simulink model "Suspension_model_PID"  (R2023a)
settings: Solver=ode1  StartTime=0.0  StopTime=10  FixedStep=0.001  RelTol=1e-3
undefined symbols (not defined in the file or in its folder): A, B, C, D, k
libraries: slpidlib x1
settings Model: Creator=ku53058  LastModifiedBy=sevva
settings SolverCC: AlgebraicLoopSolver=TrustRegion
settings DataIOCC: ReturnWorkspaceOutputs=off
settings OptimizationCC: LifeSpan=inf
settings DebuggingCC: UnconnectedInputMsg=warning  UnconnectedOutputMsg=warning  UnconnectedLineMsg=warning  ArithmeticOperatorsInVariantConditions=warning
settings ModelReferenceCC: EnableRefExpFcnMdlSchedulingChecks=on
settings SFSimCC: SimUseLocalCustomCode=off  CustomCodeUndefinedFunction=UseInterfaceOnly
settings RTWCC: RTWUseLocalCustomCode=off
settings CodeAppCC: StateflowObjectComments=on

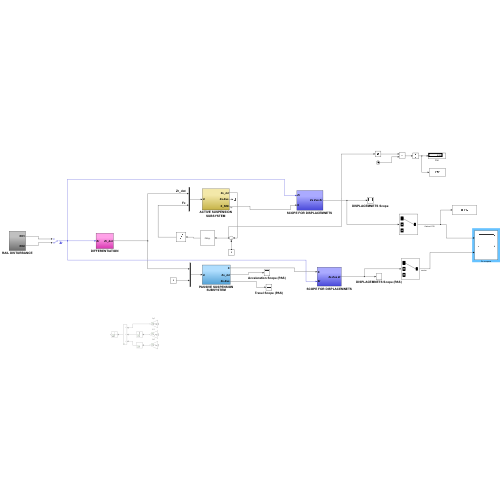
[thumbnail: Simulink's stored preview of the top-level diagram]
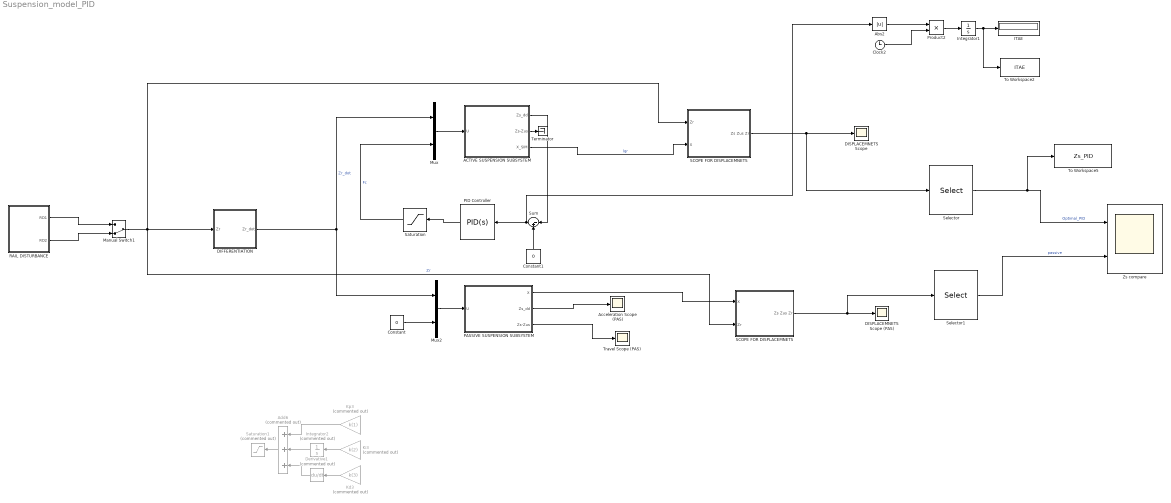
== system Suspension_model_PID ==
  ACTIVE SUSPENSION SUBSYSTEM : Subsystem
  Abs2 : Abs  SaturateOnIntegerOverflow=off
  Acceleration Scope (PAS) : Scope
  Add6 : Sum  Commented=on  Inputs=+++
  Clock2 : Clock
  Constant : Constant  Value=0
  Constant1 : Constant  Value=0
  DIFFERENTIATION : Subsystem
  DISPLACEMNETS Scope : Scope
  DISPLACEMNETS Scope (PAS) : Scope
  Derivative1 : Derivative  Commented=on
  ITAE : Display
  Integrator1 : Integrator
  Integrator2 : Integrator  Commented=on
  Kd3 : Gain  Commented=on  Gain=k(3)
  Ki3 : Gain  Commented=on  Gain=k(2)
  Kp3 : Gain  Commented=on  Gain=k(1)
  Manual Switch1 : ManualSwitch  CurrentSetting=0
  Mux : Mux  Inputs=2
  Mux2 : Mux  Inputs=2
  PASSIVE SUSPENSION SUBSYSTEM : Subsystem
  PID Controller : slpidlib/PID Controller  Controller=PID  Form=Parallel  TimeDomain=Continuous-time  UseExternalTs=off  SampleTime=-1  IntegratorMethod=Forward Euler  FilterMethod=Forward Euler  ControllerParametersSource=internal  P=150  I=3000  UseKiTs=off  D=45  N=100  UseFilter=on  TunerSelectOption=Transfer Function Based (PID Tuner App)  InitialConditionSource=internal  InitialConditionForIntegrator=0  InitialConditionForFilter=0  DifferentiatorICPrevScaledInput=0  ExternalReset=none  TrackingMode=off  Kt=1  LimitOutput=off  SatLimitsSource=internal  UpperSaturationLimit=inf  LowerSaturationLimit=-inf  LinearizeAsGain=on  AntiWindupMode=none  Kb=1  LimitIntegrator=off  UpperIntegratorSaturationLimit=inf  LowerIntegratorSaturationLimit=-inf  POutMin=[]  POutMax=[]  IOutMin=[]  IOutMax=[]  DOutMin=[]  DOutMax=[]  NOutMin=[]  NOutMax=[]  SumOutMin=[]  SumOutMax=[]  SaturationOutMin=[]  SaturationOutMax=[]  PParamMin=[]  PParamMax=[]  IParamMin=[]  IParamMax=[]  DParamMin=[]  DParamMax=[]  NParamMin=[]  NParamMax=[]  KbParamMin=[]  KbParamMax=[]  KtParamMin=[]  KtParamMax=[]  KbOutMin=[]  KbOutMax=[]  KtOutMin=[]  KtOutMax=[]  IntegratorOutMin=[]  IntegratorOutMax=[]  FilterOutMin=[]  FilterOutMax=[]  SumI1OutMin=[]  SumI1OutMax=[]  SumI2OutMin=[]  SumI2OutMax=[]  SumI3OutMin=[]  SumI3OutMax=[]  SumI4OutMin=[]  SumI4OutMax=[]  SumDOutMin=[]  SumDOutMax=[]  DifferentiatorOutMin=[]  DifferentiatorOutMax=[]  FilterDiffOutCoefMin=[]  FilterDiffOutCoefMax=[]  ReciprocalOutMin=[]  ReciprocalOutMax=[]  SumDenOutMin=[]  SumDenOutMax=[]  SumNumOutMin=[]  SumNumOutMax=[]  DivideOutMin=[]  DivideOutMax=[]  UdiffTsProdOutMin=[]  UdiffTsProdOutMax=[]  NTsProdOutMin=[]  NTsProdOutMax=[]  UintegralTsProdOutMin=[]  UintegralTsProdOutMax=[]  UngainTsProdOutMin=[]  UngainTsProdOutMax=[]  ClampingZeroOutDataTypeStr=Inherit: Inherit via back propagation  ClampingZeroOutMin=[]  ClampingZeroOutMax=[]  FilterDenConstantOutDataTypeStr=Inherit: Inherit via back propagation  FilterDenConstantOutMin=[]  FilterDenConstantOutMax=[]  PCopyOutDataTypeStr=Inherit: Inherit via back propagation  PCopyOutMin=[]  PCopyOutMax=[]  NCopyOutDataTypeStr=Inherit: Inherit via back propagation  NCopyOutMin=[]  NCopyOutMax=[]  IntegratorContinuousStateAttributes=''  IntegratorStateMustResolveToSignalObject=off  IntegratorRTWStateStorageClass=Auto  FilterContinuousStateAttributes=''  FilterStateMustResolveToSignalObject=off  FilterRTWStateStorageClass=Auto  ParallelPVariant=InternalParameters  IdealPVariant=Disabled  IVariant=InternalParameters  DVariant=InternalParameters  IntegratorVariant=Continuous  SatVariant=Disabled  AWVariant=Passthrough  PCopyVariant=Disabled  TRVariant=Disabled  FdbkBlocksVariant=Forward  IdealPFdbkVariant=Disabled  SatFdbkVariant=Disabled  DerivativeFilterVariant=ContFilter  NVariant=InternalParameters  NCopyVariant=Disabled  FilterICVariant=InternalICsFilter  IntegratorICVariant=InternalICs  ExternalResetVariant=Disabled  TRSumVariant=Passthrough  SumFdbkVariant=Disabled  SumVariant=Sum_PID  TsampFilterVariant=InternalTs  TsampNgainVariant=Passthrough  TsampIntegralVariant=Disabled_SignalSpec  ExternalSaturationOutDataTypeStr=Inherit: Same as second input
  Product2 : Product
  RAIL DISTURBANCE : Subsystem
  SCOPE FOR DISPLACEMNETS : Subsystem
  "SCOPE FOR DISPLACEMNETS " : Subsystem
  Saturation : Saturate  UpperLimit=46730  LowerLimit=-46730
  Saturation1 : Saturate  Commented=on  UpperLimit=46730  LowerLimit=-46730
  Selector : Selector  InputPortWidth=3  IndexOptions=Index vector (dialog)  Indices=[1]  OutputSizes=1
  Selector1 : Selector  InputPortWidth=3  IndexOptions=Index vector (dialog)  Indices=[1]  OutputSizes=1
  Sum : Sum  Inputs=|-+
  Terminator : Terminator
  To Workspace2 : ToWorkspace  VariableName=ITAE  SampleTime=-1
  To Workspace5 : ToWorkspace  VariableName=Zs_PID  SaveFormat=Timeseries  SampleTime=-1
  Travel Scope (PAS) : Scope
  Zs compare : Scope  NumInputPorts=2
  wires:
  PID Controller/1 -> Saturation/1
  Constant/1 -> Mux2/2
  Saturation/1 -> Mux/2  "Fc"
  Mux/1 -> ACTIVE SUSPENSION SUBSYSTEM/1(U)
  "SCOPE FOR DISPLACEMNETS "/1(Zs Zus Zr) -> Selector/1, DISPLACEMNETS Scope/1
  Mux2/1 -> PASSIVE SUSPENSION SUBSYSTEM/1(U)
  PASSIVE SUSPENSION SUBSYSTEM/1(X) -> SCOPE FOR DISPLACEMNETS/1(X)
  SCOPE FOR DISPLACEMNETS/1(Zs Zus Zr) -> Selector1/1, DISPLACEMNETS Scope (PAS)/1
  PASSIVE SUSPENSION SUBSYSTEM/2(Zs_dd) -> Acceleration Scope (PAS)/1
  PASSIVE SUSPENSION SUBSYSTEM/3(Zs-Zus) -> Travel Scope (PAS)/1
  RAIL DISTURBANCE/1(RD1) -> Manual Switch1/1
  RAIL DISTURBANCE/2(RD2) -> Manual Switch1/2
  Selector/1 -> To Workspace5/1, Zs compare/1  "Optimal_PID"
  DIFFERENTIATION/1(Zr_dot) -> Mux2/1, Mux/1  "Zr_dot"
  Manual Switch1/1 -> SCOPE FOR DISPLACEMNETS/2(Zr), DIFFERENTIATION/1(Zr), "SCOPE FOR DISPLACEMNETS "/1(Zr)  "Zr"
  Selector1/1 -> Zs compare/2  "passive"
  ACTIVE SUSPENSION SUBSYSTEM/1(Zs_dd) -> Sum/1
  Constant1/1 -> Sum/2
  ACTIVE SUSPENSION SUBSYSTEM/3(X_SIM) -> "SCOPE FOR DISPLACEMNETS "/2(X)  "lqr"
  Product2/1 -> Integrator1/1
  Abs2/1 -> Product2/1
  Clock2/1 -> Product2/2
  Integrator1/1 -> To Workspace2/1, ITAE/1
  Add6/1 -> Saturation1/1
  Ki3/1 -> Integrator2/1
  Kp3/1 -> Add6/1
  Derivative1/1 -> Add6/3
  Sum/1 -> PID Controller/1, Abs2/1
  Kd3/1 -> Derivative1/1
  Integrator2/1 -> Add6/2
  ACTIVE SUSPENSION SUBSYSTEM/2(Zs-Zus) -> Terminator/1

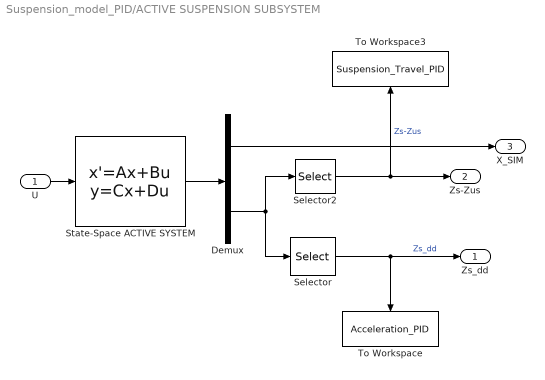
== system Suspension_model_PID/ACTIVE SUSPENSION SUBSYSTEM ==
  U : Inport
  Demux : Demux  Outputs=[4 2]
  Selector : Selector  InputPortWidth=2  IndexOptions=Index vector (dialog)  Indices=[2]  OutputSizes=1
  Selector2 : Selector  InputPortWidth=2  IndexOptions=Index vector (dialog)  Indices=[1]  OutputSizes=1
  State-Space ACTIVE SYSTEM : StateSpace  A=A  B=B  C=cat(1,eye(4), C)  D=D  InitialCondition=0
  To Workspace : ToWorkspace  VariableName=Acceleration_PID  SaveFormat=Timeseries  SampleTime=-1
  To Workspace3 : ToWorkspace  VariableName=Suspension_Travel_PID  SaveFormat=Timeseries  SampleTime=-1
  Zs_dd : Outport
  Zs-Zus : Outport  Port=2
  X_SIM : Outport  Port=3
  wires:
  Demux/1 -> X_SIM/1
  State-Space ACTIVE SYSTEM/1 -> Demux/1
  Demux/2 -> Selector2/1, Selector/1
  Selector/1 -> Zs_dd/1, To Workspace/1  "Zs_dd"
  Selector2/1 -> Zs-Zus/1, To Workspace3/1  "Zs-Zus"
  U/1 -> State-Space ACTIVE SYSTEM/1

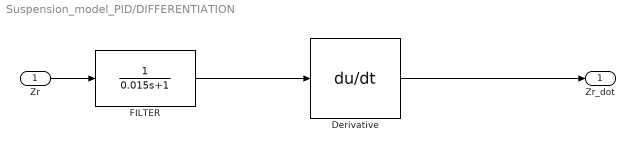
== system Suspension_model_PID/DIFFERENTIATION ==
  Zr : Inport
  Derivative : Derivative
  FILTER : TransferFcn  Denominator=[0.015 1]
  Zr_dot : Outport
  wires:
  FILTER/1 -> Derivative/1
  Derivative/1 -> Zr_dot/1
  Zr/1 -> FILTER/1

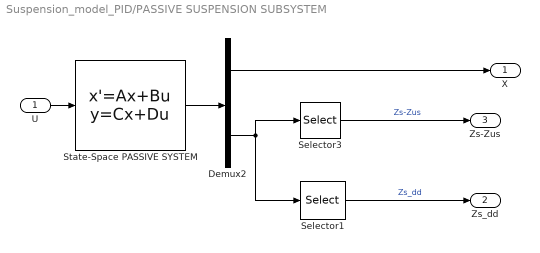
== system Suspension_model_PID/PASSIVE SUSPENSION SUBSYSTEM ==
  U : Inport
  Demux2 : Demux  Outputs=[4 2]
  Selector1 : Selector  InputPortWidth=2  IndexOptions=Index vector (dialog)  Indices=[2]  OutputSizes=1
  Selector3 : Selector  InputPortWidth=2  IndexOptions=Index vector (dialog)  Indices=[1]  OutputSizes=1
  State-Space PASSIVE SYSTEM : StateSpace  A=A  B=B  C=cat(1,eye(4), C)  D=D  InitialCondition=0
  X : Outport
  Zs_dd : Outport  Port=2
  Zs-Zus : Outport  Port=3
  wires:
  State-Space PASSIVE SYSTEM/1 -> Demux2/1
  Selector1/1 -> Zs_dd/1  "Zs_dd"
  Demux2/2 -> Selector3/1, Selector1/1
  Selector3/1 -> Zs-Zus/1  "Zs-Zus"
  U/1 -> State-Space PASSIVE SYSTEM/1
  Demux2/1 -> X/1

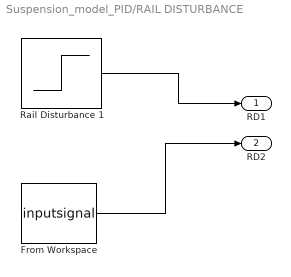
== system Suspension_model_PID/RAIL DISTURBANCE ==
  From Workspace : FromWorkspace  VariableName=inputsignal
  Rail Disturbance 1 : Step  After=0.06  SampleTime=0
  RD1 : Outport
  RD2 : Outport  Port=2
  wires:
  From Workspace/1 -> RD2/1
  Rail Disturbance 1/1 -> RD1/1

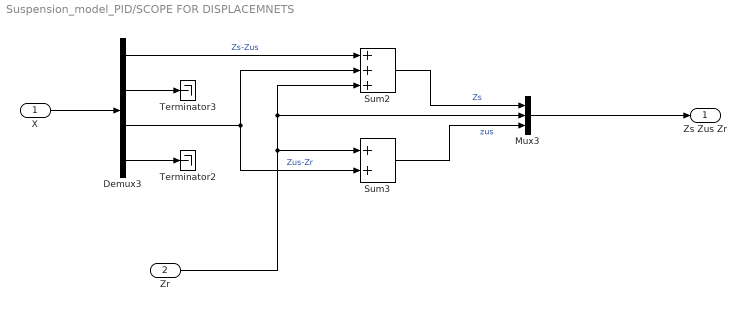
== system Suspension_model_PID/SCOPE FOR DISPLACEMNETS ==
  X : Inport
  Zr : Inport  Port=2
  Demux3 : Demux
  Mux3 : Mux  Inputs=3
  Sum2 : Sum  Inputs=+++
  Sum3 : Sum
  Terminator2 : Terminator
  Terminator3 : Terminator
  Zs Zus Zr : Outport
  wires:
  Demux3/2 -> Terminator3/1
  Demux3/4 -> Terminator2/1
  Demux3/1 -> Sum2/1  "Zs-Zus"
  Demux3/3 -> Sum3/2, Sum2/2  "Zus-Zr"
  Sum2/1 -> Mux3/1  "Zs"
  Sum3/1 -> Mux3/3  "zus"
  Mux3/1 -> Zs Zus Zr/1
  Zr/1 -> Sum3/1, Mux3/2, Sum2/3
  X/1 -> Demux3/1

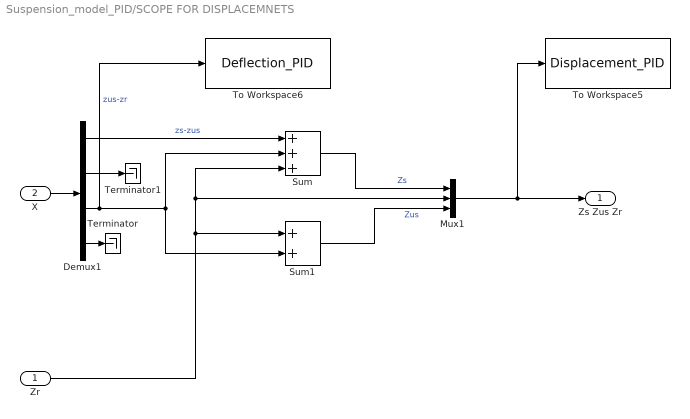
== system Suspension_model_PID/SCOPE FOR DISPLACEMNETS  ==
  Zr : Inport
  X : Inport  Port=2
  Demux1 : Demux
  Mux1 : Mux  Inputs=3
  Sum : Sum  Inputs=+++
  Sum1 : Sum
  Terminator : Terminator
  Terminator1 : Terminator
  To Workspace5 : ToWorkspace  VariableName=Displacement_PID  SaveFormat=Timeseries  SampleTime=-1
  To Workspace6 : ToWorkspace  VariableName=Deflection_PID  SaveFormat=Timeseries  SampleTime=-1
  Zs Zus Zr : Outport
  wires:
  X/1 -> Demux1/1
  Demux1/2 -> Terminator1/1
  Demux1/4 -> Terminator/1
  Demux1/1 -> Sum/1  "zs-zus"
  Demux1/3 -> To Workspace6/1, Sum1/2, Sum/2  "zus-zr"
  Sum/1 -> Mux1/1  "Zs"
  Sum1/1 -> Mux1/3  "Zus"
  Mux1/1 -> Zs Zus Zr/1, To Workspace5/1
  Zr/1 -> Sum1/1, Mux1/2, Sum/3
